simulink model "CUK_Converter (2)"  (R2024a)
settings: Solver=VariableStepAuto  StartTime=0.0  StopTime=10.0  RelTol=1e-3
libraries: spsCurrentMeasurementLib x7, spsVoltageMeasurementLib x7, spsSeriesRLCBranchLib x6, spsDCVoltageSourceLib x1, spsDiodeLib x1, spsMosfetLib x1, sps_lib x1
settings Model: Creator=Saharsh  LastModifiedBy=Saharsh

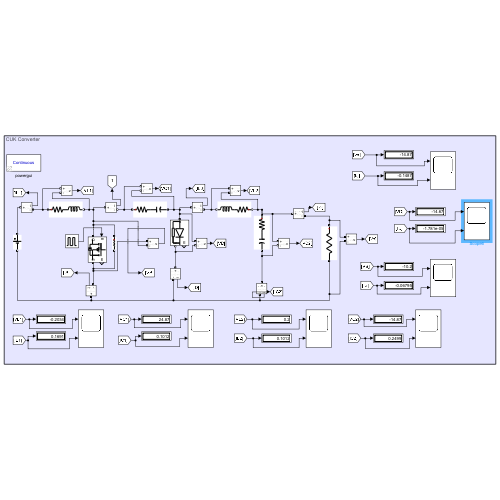
[thumbnail: Simulink's stored preview of the top-level diagram]
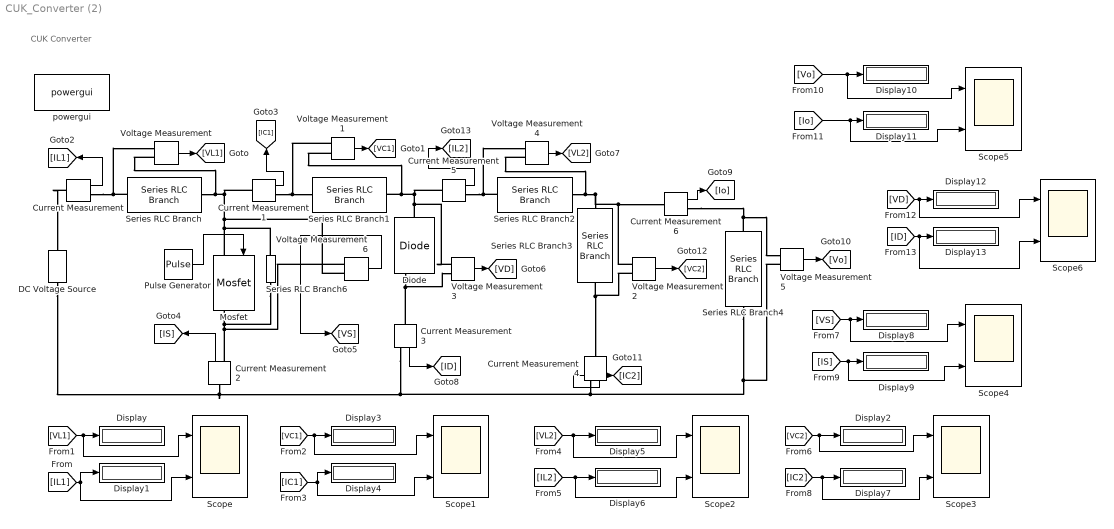
== system CUK_Converter (2) ==
  note: CUK Converter
  Current Measurement{,1..6} (7 alike) : spsCurrentMeasurementLib/Current Measurement  PhasorSimulation=off  OutputType=Complex  PSBequivalent=0
  DC Voltage Source : spsDCVoltageSourceLib/DC Voltage Source  Amplitude=10  Measurements=None
  Diode : spsDiodeLib/Diode  Ron=0.01  Lon=0  Vf=1.8  IC=0  UseSnubber=0  Rs=500  Cs=250e-12  Measurements=on
  Display{,1..13} (14 alike) : Display
  Mosfet : spsMosfetLib/Mosfet  Ron=0.05  Lon=0  Rd=0.0175  Vfd=0.8  IC=0  Rs=150  Cs=1e-9  Measurements=on
  Pulse Generator : DiscretePulseGenerator  PulseType=Time based  Amplitude=12  Period=1e-4  PulseWidth=56.45
  Scope{,1..6} (7 alike) : Scope  NumInputPorts=2
  Series RLC Branch : spsSeriesRLCBranchLib/Series RLC Branch  LConnTagsString=__new0  RConnTagsString=__new0  BranchType=RL  Resistance=0.25  Inductance=1e-3  SetiL0=off  InitialCurrent=0  Capacitance=1e-6  Setx0=off  InitialVoltage=0  Measurements=None
  Series RLC Branch1 : spsSeriesRLCBranchLib/Series RLC Branch  LConnTagsString=__new0  RConnTagsString=__new0  BranchType=RC  Resistance=0.2  Inductance=1e-3  SetiL0=off  InitialCurrent=0  Capacitance=100e-6  Setx0=off  InitialVoltage=0  Measurements=None
  Series RLC Branch2 : spsSeriesRLCBranchLib/Series RLC Branch  LConnTagsString=__new0  RConnTagsString=__new0  BranchType=RL  Resistance=0.25  Inductance=1e-3  SetiL0=off  InitialCurrent=0  Capacitance=1e-6  Setx0=off  InitialVoltage=0  Measurements=None
  Series RLC Branch3 : spsSeriesRLCBranchLib/Series RLC Branch  LConnTagsString=__new0  RConnTagsString=__new0  BranchType=RC  Resistance=0.08  Inductance=1e-3  SetiL0=off  InitialCurrent=0  Capacitance=470e-6  Setx0=off  InitialVoltage=0  Measurements=None
  Series RLC Branch4 : spsSeriesRLCBranchLib/Series RLC Branch  LConnTagsString=__new0  RConnTagsString=__new0  BranchType=R  Resistance=100  Inductance=1e-3  SetiL0=off  InitialCurrent=0  Capacitance=1e-6  Setx0=off  InitialVoltage=0  Measurements=None
  Series RLC Branch6 : spsSeriesRLCBranchLib/Series RLC Branch  LConnTagsString=__new0  RConnTagsString=__new0  BranchType=R  Resistance=150  Inductance=1e-3  SetiL0=off  InitialCurrent=0  Capacitance=1e-6  Setx0=off  InitialVoltage=0  Measurements=None
  Voltage Measurement{,1..6} (7 alike) : spsVoltageMeasurementLib/Voltage Measurement  PhasorSimulation=off  OutputType=Complex  PSBequivalent=0
  powergui : sps_lib/powergui  Priority=1  SimulationMode=Continuous  SampleTime=50e-6  frequency=60  Iterations=50  frequencyindice=0  Pbase=100e6  ErrMax=1e-4  UnitsV=kV  UnitsW=MW  buscounter=0  FunctionMessages=off  echomessages=off  EnableUseOfTLC=off  CurrentSourceSwitches=off  DisableSnubberDevices=off  DisableRonSwitches=off  DisableVfSwitches=off  DisplayEquations=off  AutomaticDiscreteSolvers=off  SolverType=Tustin/Backward Euler (TBE)  Interpol=off  ExternalGateDelay=off  methode=off  Ts=100  x0status=blocks  SPID=on  SwTol=0  HookPort=off  NonlinearTolerance=1e-4  nMaxIteration=100  ContinueOnMaxIteration=off  RestoreLinks=warning  ResistiveCurrentMeasurement=off  Frange=[0:2:500]  Ylog=off  Xlog=on  ShowGrid=off  save=off  variable=ZData  structure=0  ZoomFFT=off  StartTime=0.0  cycles=1  DisplayStyle=1  fundamental=60  FreqAxis=off  MaxFrequency=1000  frequencyindicesteady=1  RmsSteady=1  display=off
  wires:
  Pulse Generator/1 -> Mosfet/1
  Voltage Measurement/1 -> [VL1]
  Voltage Measurement1/1 -> [VC1]
  Current Measurement/1 -> [IL1]
  Current Measurement1/1 -> [IC1]
  Current Measurement2/1 -> [IS]
  Voltage Measurement6/1 -> [VS]
  Voltage Measurement3/1 -> [VD]
  Voltage Measurement4/1 -> [VL2]
  Current Measurement3/1 -> [ID]
  Voltage Measurement5/1 -> [Vo]
  Current Measurement6/1 -> [Io]
  Voltage Measurement2/1 -> [VC2]
  Current Measurement4/1 -> [IC2]
  Current Measurement5/1 -> [IL2]
  [VL1] -> Scope/1, Display/1
  [IL1] -> Display1/1, Scope/2
  [VC1] -> Scope1/1, Display3/1
  [IC1] -> Scope1/2, Display4/1
  [VL2] -> Scope2/1, Display5/1
  [IL2] -> Scope2/2, Display6/1
  [VC2] -> Scope3/1, Display2/1
  [IC2] -> Scope3/2, Display7/1
  [VS] -> Scope4/1, Display8/1
  [IS] -> Scope4/2, Display9/1
  [Vo] -> Scope5/1, Display10/1
  [Io] -> Scope5/2, Display11/1
  [ID] -> Scope6/2, Display13/1
  [VD] -> Scope6/1, Display12/1
  connections:
  Voltage Measurement1/LConn1 -- Current Measurement1/RConn1 -- Series RLC Branch1/LConn1
  Diode/LConn1 -- Voltage Measurement3/LConn1 -- Current Measurement5/LConn1 -- Series RLC Branch1/RConn1 -- Voltage Measurement1/LConn2
  Series RLC Branch/LConn1 -- Current Measurement/RConn1 -- Voltage Measurement/LConn1
  DC Voltage Source/LConn1 -- Current Measurement2/LConn1 -- Current Measurement4/RConn1 -- Series RLC Branch4/RConn1 -- Voltage Measurement5/LConn2 -- Current Measurement3/RConn1
  Voltage Measurement4/LConn2 -- Series RLC Branch2/LConn1 -- Current Measurement6/LConn1 -- Voltage Measurement2/LConn1 -- Series RLC Branch3/LConn1
  Current Measurement/LConn1 -- DC Voltage Source/RConn1
  Voltage Measurement/LConn2 -- Series RLC Branch6/LConn1 -- Mosfet/LConn1 -- Voltage Measurement6/LConn2 -- Current Measurement1/LConn1 -- Series RLC Branch/RConn1
  Current Measurement2/RConn1 -- Series RLC Branch6/RConn1 -- Mosfet/RConn1 -- Voltage Measurement6/LConn1
  Diode/RConn1 -- Voltage Measurement3/LConn2 -- Current Measurement3/LConn1
  Series RLC Branch4/LConn1 -- Current Measurement6/RConn1 -- Voltage Measurement5/LConn1
  Current Measurement5/RConn1 -- Series RLC Branch2/RConn1 -- Voltage Measurement4/LConn1
  Voltage Measurement2/LConn2 -- Current Measurement4/LConn1 -- Series RLC Branch3/RConn1
